simulink model "controladorLQG_sim"  (R2017a)
settings: Solver=VariableStepAuto  StartTime=0.0  StopTime=100  RelTol=1e-3
values from neighbouring files (symbols this model uses):
  C = [0 1 0]    [controlador_LQR.m]
  sysKF = ss(A-L*C,[B L],eye(3),0*[B L])    [controlador_LQR.m]
undefined symbols (not defined in the file or in its folder): Kr
libraries: simulink x2
settings Model: Creator=Matheus  LastModifiedBy=Matheus

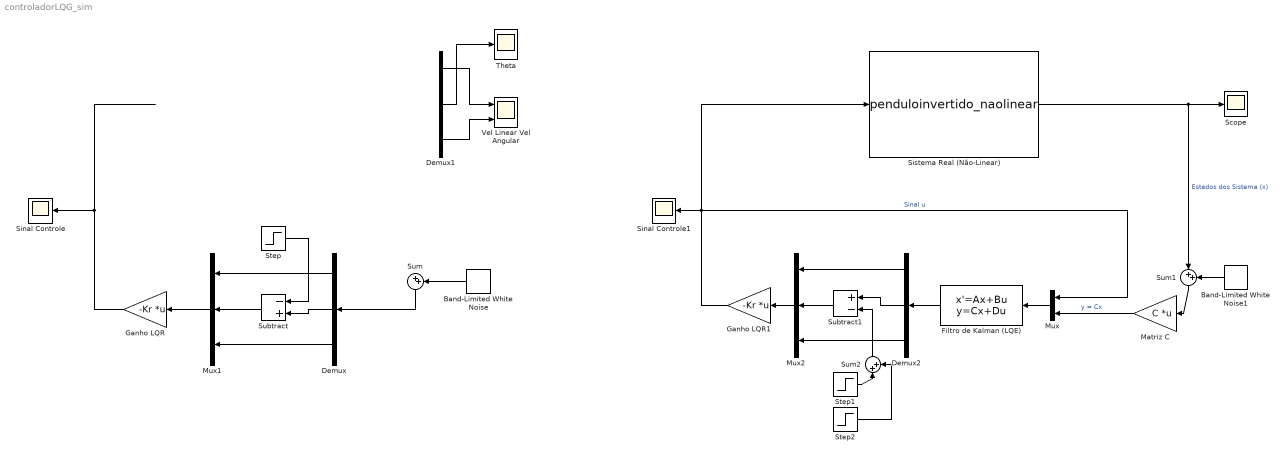
== system controladorLQG_sim ==
  Band-Limited White Noise : simulink/Sources/Band-Limited White Noise  Cov=[0]  Ts=0.1  seed=[23341]
  Band-Limited White Noise1 : simulink/Sources/Band-Limited White Noise  Cov=[0]  Ts=0.1  seed=[23341]
  Demux : Demux  Outputs=3
  Demux1 : Demux  Outputs=3
  Demux2 : Demux  Outputs=3
  Filtro de Kalman (LQE) : StateSpace  A=sysKF.a  B=sysKF.b  C=sysKF.c  D=sysKF.d  X0=[0 0 0]
  Ganho LQR : Gain  Gain=-Kr  Multiplication=Matrix(K*u) (u vector)
  Ganho LQR1 : Gain  Gain=-Kr  Multiplication=Matrix(K*u) (u vector)
  Matriz C : Gain  Gain=C  Multiplication=Matrix(K*u) (u vector)
  Mux : Mux  Inputs=2
  Mux1 : Mux  Inputs=3
  Mux2 : Mux  Inputs=3
  Scope : Scope
  Sinal Controle : Scope
  Sinal Controle1 : Scope
  Sistema Real (Não-Linear) : S-Function  InitFcn=try, set_param(gcb,'FunctionName','penduloinvertido_naolinear'), end  FunctionName=penduloinvertido_naolinear  SFunctionModules=penduloinvertido_naolinear_wrapper  SFunctionDeploymentMode=off  EnableBusSupport=off  mask(S-Function Builder){}
      mask help: Simulink:masks:SFunctionBuilder_MD
      mask init:
      | val = [[.9  0.75 0.75 1 1 .9 .9 1]',[1 1 0.75 0.75 .9 .9 1 .9]'];try , sys = get_param(gcb,'SfunBuilderFcnName');if isempty(sys), sys = get_param(gcb,'FunctionName'); end,catch, sys = get_param(gcb,'FunctionName'); end
      settings: CopyFcn=set_param(gcbh,'LinkStatus','none')  PreSaveFcn=try, set_param(gcb,'FunctionName','penduloinvertido_naolinear'), end  OpenFcn=sfunctionwizard(gcbh)
      mask Display: plot(val(:,1),val(:,2)),disp(sys), port_label('input',1,'u0'), port_label('output',1,'y0')
  Step : Step  Time=10  After=0  SampleTime=0
  Step1 : Step  Time=10  After=3.14/50  SampleTime=0
  Step2 : Step  Time=11  After=-3.14/50  SampleTime=0
  Subtract : Sum  Inputs=-+
  Subtract1 : Sum  Inputs=+-
  Sum : Sum  Inputs=|++
  Sum1 : Sum  Inputs=|++
  Sum2 : Sum  Inputs=|++
  Theta : Scope
  Vel Linear Vel Angular : Scope  NumInputPorts=2
  wires:
  Mux1/1 -> Ganho LQR/1
  ? -> Demux1/1, Sum/1
  Band-Limited White Noise/1 -> Sum/2
  Sum/1 -> Demux/1
  Demux/3 -> Mux1/3
  Ganho LQR/1 -> Sinal Controle/1
  Demux1/2 -> Theta/1
  Subtract/1 -> Mux1/2
  Step/1 -> Subtract/1
  Demux1/3 -> Vel Linear Vel Angular/2
  Demux1/1 -> Vel Linear Vel Angular/1
  Demux/2 -> Subtract/2
  Demux/1 -> Mux1/1
  Subtract1/1 -> Mux2/2
  Demux2/1 -> Mux2/1
  Mux2/1 -> Ganho LQR1/1
  Sistema Real (Não-Linear)/1 -> Scope/1, Sum1/1  "Estados dos Sistema (x)"
  Band-Limited White Noise1/1 -> Sum1/2
  Ganho LQR1/1 -> Sistema Real (Não-Linear)/1, Sinal Controle1/1, Mux/1  "Sinal u"
  Demux2/3 -> Mux2/3
  Sum1/1 -> Matriz C/1
  Filtro de Kalman (LQE)/1 -> Demux2/1
  Mux/1 -> Filtro de Kalman (LQE)/1
  Matriz C/1 -> Mux/2  "y = Cx"
  Demux2/2 -> Subtract1/1
  Step1/1 -> Sum2/1
  Step2/1 -> Sum2/2
  Sum2/1 -> Subtract1/2
